simulink model "bluetooth_voice"  (Simulink 4.1.1)
settings: Solver=VariableStepDiscrete  StartTime=0.0  StopTime=2.7  RelTol=1e-3
PreLoadFcn:
  | bluetooth_init;
values from neighbouring files (symbols this model uses):
  Access_Code = zeros(72,1); Access_Code(1:2:72)=1    [bluetooth_init.m]
  ARQ = [1]    [bluetooth_init.m]
  awgn_channel_seed = randseed(2)    [bluetooth_init.m]
  data_seed = randseed(5)    [bluetooth_init.m]
  Flow_Control = [1]    [bluetooth_init.m]
  Input_Fs = 8000    [bluetooth_init.m]
  Num_Slots_Rate = 6    [device_init.m]
  One_Zero_Payload = zeros(240,1)    [bluetooth_init.m]
  Packet_Type = [1 0 1 0]'    [bluetooth_init.m]
  Sequence = [1]    [bluetooth_init.m]
  Slave_Address = [1 0 1]'    [bluetooth_init.m]
  Slot_Enable_Phase = Slot_Pair*2-2    [device_init.m]
  Slot_Ts = (1/1600)    (= 0.000625)    [device_init.m]
  Tx_Ts = Slot_Ts*6    (= 0.00375)    [device_init.m]
undefined symbols (not defined in the file or in its folder): Fs, g, jet
libraries: commblkcod2 x48, dspsrcs3 x25, dspsigops x18, simulink3 x16, dspsigattribs x9, dspbuff3 x7, dspindex x7, bluetooth_lib x5, dspmathops x4, dspsnks3 x4, dspmtrx3 x3, commdigbbndfm2 x3
(part 1 of 2)
settings Model: Creator=Stuart McGarrity  LastModifiedBy=stuartm  SaveTime=off  SaveOutput=off  OptimizeBlockIOStorage=off  BlockReductionOpt=off
settings Model: ModifiedComment=|
  | stuartm -- Fri Jul 20 12:58:27 2001 -- Version 1.201
  | Fix for R12.1. Changed CPM modulator. Replaced enable subsystems in channel with "switch case".
settings Model: ModifiedHistory=|
  | stuartm -- Fri Jul 20 12:58:27 2001 -- Version 1.201
  | Fix for R12.1. Changed CPM modulator. Replaced enable subsystems in channel with "switch case".
  | 
  | 
  | stuartm -- Sun Jul 08 13:59:13 2001 -- Version 1.172
  | Added gain mask at output of transmitter to run it off after 374 bits.
  | 
  | stuartm -- Sun Jul 08 13:53:19 2001 -- Version 1.171
  | Changed hop generator to randint block. Put zero padiing back to before transmitter.
  | 
  | 
  | Started with bluetooth_voice2. Move zero pad from input to output of transmitter. Now only transmits 374 bits
  | 
  | Added channel option

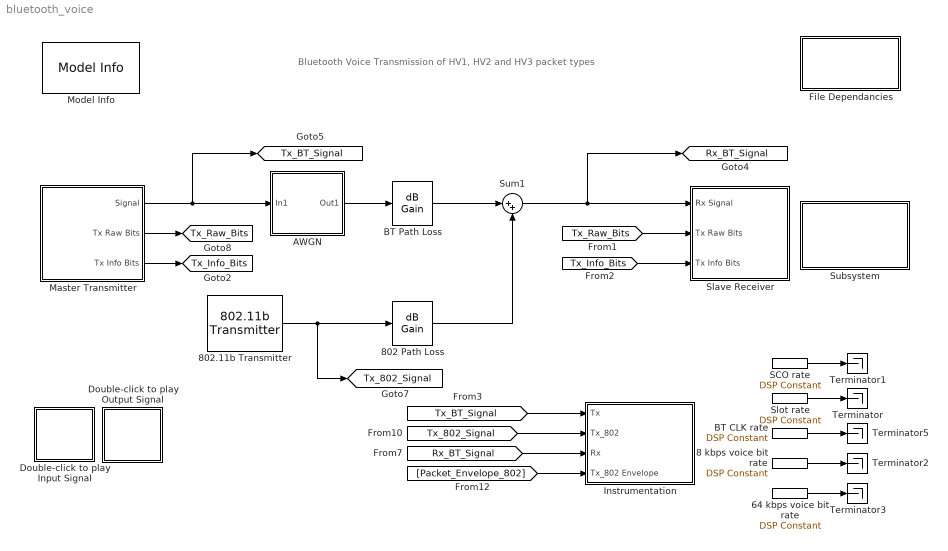
== system bluetooth_voice ==
  note: Bluetooth Voice Transmission
      | of HV1, HV2 and HV3 packet types
  64 kbps voice bit rate : dspsrcs3/DSP Constant  Value=1  InterpretAs1D=off  SampleMode=Discrete  Ts=1/64000  FramebasedOutput=off
  8 kbps voice bit rate : dspsrcs3/DSP Constant  Value=1  InterpretAs1D=off  SampleMode=Discrete  Ts=1/8000  FramebasedOutput=off
  802 Path Loss : dspmathops/dB Gain  Gain=g  dB=-40  intype=Amplitude
  802.11b Transmitter : bluetooth_lib/802.11b Transmitter  On=on  rate=200  m=1e-3  v=0  power=1  Freq_Number=39  rate_seed=rate_802_seed  awgn_seed=awgn_802_seed
  AWGN : Subsystem  TreatAsAtomicUnit=on  mask(Optional channel){AWGN_On=on, EsNo=14, Power=.001, Symbol_Period=1e-6, seed=awgn_channel_seed}
      mask prompts: AWGN_On "Turn on AWGN"; EsNo "Es/No"; Power "Input Power"; Symbol_Period "Symbol Period"
      mask init:
      | if AWGN_On==1
      |    Name='On';
      | else
      |   Name='Off';
      | end;
      settings: RTWFcnNameOpts=Auto  RTWFileNameOpts=Auto
      mask Display: disp(['AWGN is ' Name])
  BT CLK rate : dspsrcs3/DSP Constant  Value=1  InterpretAs1D=off  SampleMode=Discrete  Ts=.5/1600  FramebasedOutput=off
  BT Path Loss : dspmathops/dB Gain  Gain=g  dB=-40  intype=Amplitude
  Double-click to play Input Signal : Subsystem  mask(Plot histogram){}
      mask init:
      | [x,y,x1,y1,x2,y2] = dspblkwao2('icon');
      settings: OpenFcn=[Input_Wave,Input_Fs]=wavread('Input.wav');sound(Input_Wave,Input_Fs);  RTWFcnNameOpts=Auto  RTWFileNameOpts=Auto
      mask Display:
      | patch(x1,y1,[1 1 1]*.5);
      | patch(x2,y2);
      | plot(x,y); plot(x1,y1)
  Double-click to play Output Signal : Subsystem  mask(Plot histogram){}
      mask init:
      | [x,y,x1,y1,x2,y2] = dspblkwao2('icon');
      settings: OpenFcn=[Output_Wave,Output_Fs]=wavread('Output.wav');sound(Output_Wave,Output_Fs);  RTWFcnNameOpts=Auto  RTWFileNameOpts=Auto
      mask Display:
      | patch(x1,y1,[1 1 1]*.5);
      | patch(x2,y2);
      | plot(x,y); plot(x1,y1)
  File Dependancies : Subsystem
      settings: RTWFcnNameOpts=Auto  RTWFileNameOpts=Auto
      mask Display: disp('File\nDependancies')
  Instrumentation : Subsystem  TreatAsAtomicUnit=on  mask(Instrumentation){On=on, Off=off}
      mask init:
      | if strcmp(On,'on')
      |   string='Instrumentation\nis On\n(Double-Click\n to Toggle)\n ';
      |   set_param([gcb,'/State'],'Value','1');
      | else
      |   string='Instrumentation\nis Off\n(Double-Click\n to Toggle)\n ';
      |   set_param([gcb,'/State'],'Value','0');
      | end
      settings: OpenFcn=temp=get_param(gcb,'On');set_param(gcb,'On', get_param(gcb,'Off'));set_param(gcb,'Off', temp);  RTWFcnNameOpts=Auto  RTWFileNameOpts=Auto
      mask Display: disp(string);
  Master Transmitter : Subsystem  mask(Master Transmitter){HV_Type=HV3, Slot_Pair=1&2}
      mask prompts: HV_Type "HV Packet Type"; Slot_Pair "Initial Slot Pair for HV2 or HV3"
      mask init:
      | device_init
      settings: RTWFcnNameOpts=Auto  RTWFileNameOpts=Auto
      mask StyleString: popup(HV1|HV2|HV3),popup(1&2|3&4|5&6)
      mask Display: plot(0,0,100,100,[30,60,60,55,55,30,30],[10,10,90,90,70,70,10],[35,35,55,55,35],[64,45,45,64,64])
  Model Info : simulink3/Signals & Systems/Model Info  InitialBlockCM=none  BlockCM=none  Frame=on  DisplayStringWithTags=|  HorizontalTextAlignment=Center  LeftAlignmentValue=0.5  SourceBlockDiagram=bluetooth_voice  TagMaxNumber=20
      | Bluetooth Voice
      | %<ModelVersion>
  SCO rate : dspsrcs3/DSP Constant  Value=1  InterpretAs1D=off  SampleMode=Discrete  Ts=6/1600  FramebasedOutput=off
  Slave Receiver : Subsystem  mask(Slave Receiver){HV_Type=HV3, Slot_Pair=1&2}
      mask prompts: HV_Type "HV Packet Type"; Slot_Pair "Initial Slot Pair for HV2 or HV3"
      mask init:
      | device_init
      settings: RTWFcnNameOpts=Auto  RTWFileNameOpts=Auto
      mask StyleString: popup(HV1|HV2|HV3),popup(1&2|3&4|5&6)
      mask Display: plot(15,5,95,80,[26, 28,35,44,58,85,87,92,86,59,46,46,38, 31, 27,26],[55,49,45,45,34,15,10,16,17,37,50,58,66,67,62,55],[32,34,37,42,46,46],[67,69,71,70,66,58],[27,25,24,21,23,26],[52,49,45,47,52,58],[35,38,40,42,44],[66,67,66,64,61],[34,32,38,40,34],[60,56,51,55,60])
  Slot rate : dspsrcs3/DSP Constant  Value=1  InterpretAs1D=off  SampleMode=Discrete  Ts=1/1600  FramebasedOutput=off
  Subsystem : Subsystem
      settings: OpenFcn=open_system([bdroot '/Slave Receiver/Demodulate and decode'])  RTWFcnNameOpts=Auto  RTWFileNameOpts=Auto
      mask Display: disp('Double-click to open\n subsystem with\nBER meters\ninside receiver')
  Sum1 : Sum  Inputs=|++  SaturateOnIntegerOverflow=on
  Terminator{,1..3,5} (5 alike) : Terminator
  tag scope: Rx_BT_Signal=global, Tx_802_Signal=global, Tx_BT_Signal=global, Tx_Info_Bits=global, Tx_Raw_Bits=global
  wires:
  Master Transmitter/1(Signal) -> [Tx_BT_Signal], AWGN/1(In1)
  Sum1/1 -> [Rx_BT_Signal], Slave Receiver/1(Rx Signal)
  Master Transmitter/2(Tx Raw Bits) -> [Tx_Raw_Bits]
  Slot rate/1 -> Terminator/1
  SCO rate/1 -> Terminator1/1
  [Tx_Raw_Bits] -> Slave Receiver/2(Tx Raw Bits)
  64 kbps voice bit rate/1 -> Terminator3/1
  BT CLK rate/1 -> Terminator5/1
  Master Transmitter/3(Tx Info Bits) -> [Tx_Info_Bits]
  [Tx_Info_Bits] -> Slave Receiver/3(Tx Info Bits)
  8 kbps voice bit rate/1 -> Terminator2/1
  802.11b Transmitter/1 -> [Tx_802_Signal], 802 Path Loss/1
  802 Path Loss/1 -> Sum1/2
  AWGN/1(Out1) -> BT Path Loss/1
  BT Path Loss/1 -> Sum1/1
  [Tx_BT_Signal] -> Instrumentation/1(Tx)
  [Rx_BT_Signal] -> Instrumentation/3(Rx)
  [Tx_802_Signal] -> Instrumentation/2(Tx_802)
  [Packet_Envelope_802] -> Instrumentation/4(Tx_802 Envelope)

== system bluetooth_voice/AWGN ==
  In1 : Inport  Port=1  LatchInput=off
  Generate noise only for slot 1 : simulink3/Nonlinear/Manual Switch  sw=0  action=0
  Mode : Constant  Value=AWGN_On
  Slot 1 enable2 : dspsrcs3/Signal From Workspace  X=[1 0 0 0 0 0]  Ts=625e-6  nsamps=1  OutputAfterFinalValue=Cyclic Repetition
  Slot 1 enable3 : dspsrcs3/Signal From Workspace  X=[1 1 1 1 1 1 ]  Ts=625e-6  nsamps=1  OutputAfterFinalValue=Cyclic Repetition
  Subsystem : Subsystem  TreatAsAtomicUnit=on
      settings: RTWFcnNameOpts=Auto  RTWFileNameOpts=Auto
  Out1 : Outport  Port=1  InitialOutput=0
  wires:
  Mode/1 -> Subsystem/1(In1)
  Subsystem/1(Out1) -> Out1/1
  Slot 1 enable3/1 -> Generate noise only for slot 1/2
  Generate noise only for slot 1/1 -> Subsystem/Enable
  Slot 1 enable2/1 -> Generate noise only for slot 1/1
  In1/1 -> Subsystem/2(In2)

== system bluetooth_voice/Double-click to play Input Signal ==

== system bluetooth_voice/Double-click to play Output Signal ==

== system bluetooth_voice/File Dependancies ==
  note: * bluetooth_init.m: Workspace initialization routine called by PreLoadFcn
      | * device_init.m: Transmitter and receiver mask initialization function
      | * bluetooth_lib.mld: Simuink library containing 802.11b transmitter, BT hop generator and BT clock
      | * poiss_gaus_pr3.m: Variable time-step M Code S-function to generate 802.11b possion packets
      | * scondemohecgen.c: S-Function builder source for HEC
      | * scondemohecgen.dll: S-Function builder DLL
      | * scondemohecgen_wrapper.c: S-Function support file
      | * Input.wav: Input wave file
      | * Output.wav: Output wave file
  note: File dependancies: These files need to on MATLAB path

== system bluetooth_voice/Instrumentation ==
  Tx : Inport  Port=1  LatchInput=off
  Tx_802 : Inport  Port=2  LatchInput=off
  Rx : Inport  Port=3  LatchInput=off
  Tx_802 Envelope : Inport  Port=4  LatchInput=off
  802.11 Packets  Transmitted : Display
      settings: Format=short
  Counter : dspswit3/Counter  Direction=Up  CountEvent=Rising edge  CounterSize=User defined  MaxCount=1000  InitialCount=0  Output=Count  HitValue=32  ResetInput=off  SamplesPerFrame=1  Ts=1
  State : Constant  Value=1
  Subsystem : Subsystem  TreatAsAtomicUnit=on
      settings: RTWFcnNameOpts=Auto  RTWFileNameOpts=Auto
  To Workspace : ToWorkspace  VariableName=Num_802_packets  SampleTime=-1  SaveFormat=Array
      settings: MaxDataPoints=1
  wires:
  Counter/1 -> To Workspace/1, 802.11 Packets  Transmitted/1
  State/1 -> Subsystem/Enable
  Tx_802 Envelope/1 -> Counter/1
  Tx_802/1 -> Subsystem/2(In2)
  Tx/1 -> Subsystem/1(In1)
  Rx/1 -> Subsystem/3(In3)

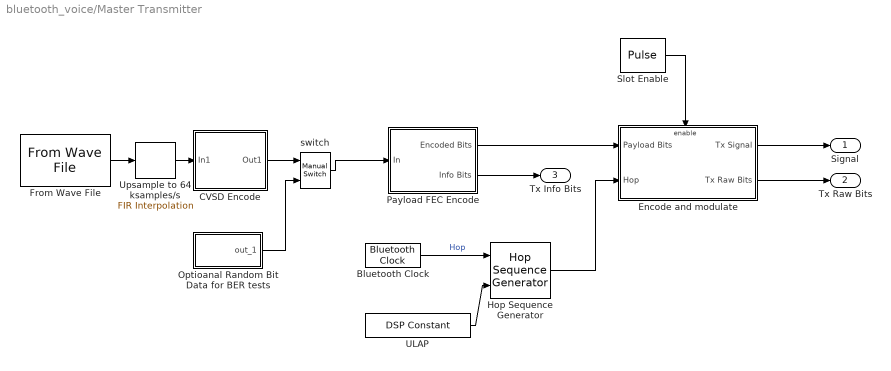
== system bluetooth_voice/Master Transmitter ==
  Bluetooth Clock : bluetooth_lib/Bluetooth Clock  Ts=(1/1600)/2
  CVSD Encode : Subsystem  mask(CVSD Encoder){min_step=10, max_step=1280, accum_decay=1-1/32, step_decay=1-1/1024}
      mask prompts: min_step "Minimum Step Size"; max_step "Maximum Step Size"; accum_decay "Accumulator Decay"; step_decay "Step Decay"
      mask help: Encode a 64 K samples per sec speech signal into a 64Kbps bit stream.
      mask init:
      | pos_accum_max = 2^15 - 1;
      | neg_accum_max = -2^15 + 1;
      settings: RTWFcnNameOpts=Auto  RTWFileNameOpts=Auto
      mask Display: disp('CVSD\nEncode')
  Encode and modulate : Subsystem  TreatAsAtomicUnit=on
      settings: RTWFcnNameOpts=Auto  RTWFileNameOpts=Auto
  From Wave File : dspsrcs3/From Wave File  FileName=Input.wav  SamplesPerFrame=1  MinBufSize=256
  Hop Sequence Generator : bluetooth_lib/Hop Sequence Generator  Hop_Mode=Connection State Hop Sequence  hop_seed=hop_seed  fixed_hop_freq=fixed_hop_freq
  Optioanal Random Bit Data for BER tests : Subsystem  mask(Random-Integer Generator){mul=2, seed=data_seed, Ts=1/64000, frameBased=off, sampPerFrame=1, orient=off}
      mask prompts: mul "M-ary number:"; seed "Initial seed:"; Ts "Sample time:"; frameBased "Frame-based outputs"; sampPerFrame "Samples per frame:"; orient "Interpret vector parameters as 1-D"
      mask help: Generate integers randomly distributed in range [0, M-1], where M is the M-ary number.
      mask init:
      | if (frameBased & sampPerFrame > 1), dsp_sampFrame = sampPerFrame;
      | else dsp_sampFrame = 1; end
      | eStr=commblkrandintsrc2(gcb,'init');
      | if(eStr.ecode==1)
      |     error(eStr.emsg);
      | end
      settings: RTWFcnNameOpts=Auto  RTWFileNameOpts=Auto
      mask Help: helpview(commbhelp)
      mask CallbackString: |||commblkrandintsrc2(gcb,'cbFrameBased');||commblkrandintsrc2(gcb,'cbOrient');
      mask Display: disp('Random bits')
  Payload FEC Encode : Subsystem
      settings: RTWFcnNameOpts=Auto  RTWFileNameOpts=Auto
  Slot Enable : DiscretePulseGenerator  PulseType=Sample-based  Amplitude=1  Period=Num_Slots_Rate  PulseWidth=1  PhaseDelay=Slot_Enable_Phase  SampleTime=Slot_Ts
  ULAP : dspsrcs3/DSP Constant  Value=hex2dec('2a96ef25')  InterpretAs1D=off  SampleMode=Discrete  Ts=(1/1600)/2  FramebasedOutput=off
  Upsample to 64 ksamples/s : dspmlti3/FIR Interpolation  h=interp_coeffs  L=8  framing=Maintain input frame size  outputBufInitCond=0
  switch : simulink3/Nonlinear/Manual Switch  sw=1  action=0
  Signal : Outport  Port=1
  Tx Raw Bits : Outport  Port=2
  Tx Info Bits : Outport  Port=3
  wires:
  Slot Enable/1 -> Encode and modulate/Enable
  Encode and modulate/1(Tx Signal) -> Signal/1
  Payload FEC Encode/1(Encoded Bits) -> Encode and modulate/1(Payload Bits)
  From Wave File/1 -> Upsample to 64 ksamples/s/1
  Upsample to 64 ksamples/s/1 -> CVSD Encode/1(In1)
  Payload FEC Encode/2(Info Bits) -> Tx Info Bits/1
  Encode and modulate/2(Tx Raw Bits) -> Tx Raw Bits/1
  Hop Sequence Generator/1 -> Encode and modulate/2(Hop)
  ULAP/1 -> Hop Sequence Generator/2
  Bluetooth Clock/1 -> Hop Sequence Generator/1  "Hop"
  Optioanal Random Bit Data for BER tests/1(out_1) -> switch/2
  CVSD Encode/1(Out1) -> switch/1
  switch/1 -> Payload FEC Encode/1(In)

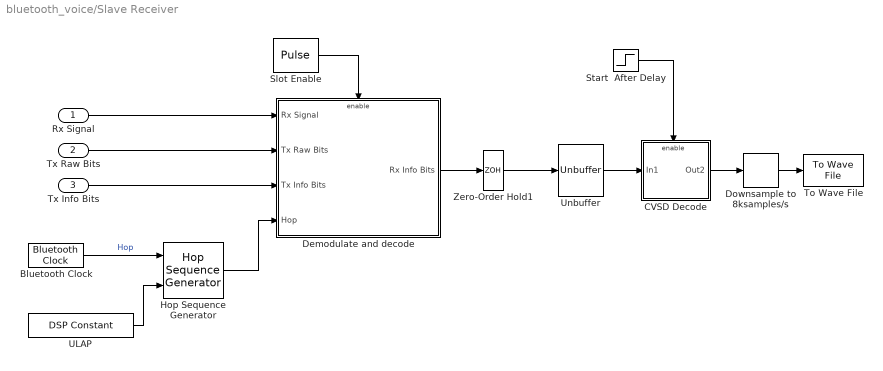
== system bluetooth_voice/Slave Receiver ==
  Rx Signal : Inport  Port=1  LatchInput=off
  Tx Raw Bits : Inport  Port=2  LatchInput=off
  Tx Info Bits : Inport  Port=3  LatchInput=off
  Bluetooth Clock : bluetooth_lib/Bluetooth Clock  Ts=(1/1600)/2
  CVSD Decode : Subsystem  TreatAsAtomicUnit=on  mask(CVSD Decoder){min_step=10, max_step=1280, accum_decay=1-1/32, step_decay=1-1/1024}
      mask prompts: min_step "Minimum Step Size"; max_step "Maximum Step Size"; accum_decay "Accumulator Decay"; step_decay "Step Decay"
      mask init:
      | pos_accum_max = 2^15 - 1;
      | neg_accum_max = -2^15 + 1;
      settings: RTWFcnNameOpts=Auto  RTWFileNameOpts=Auto
      mask Display: disp('CVSD\nDecoder')
  Demodulate and decode : Subsystem  TreatAsAtomicUnit=on
      settings: RTWFcnNameOpts=Auto  RTWFileNameOpts=Auto
  Downsample to 8ksamples/s : dspsigops/Downsample  N=8  phase=0  ic=0  smode=Allow multirate  fmode=Maintain input frame size
  Hop Sequence Generator : bluetooth_lib/Hop Sequence Generator  Hop_Mode=Connection State Hop Sequence  hop_seed=hop_seed  fixed_hop_freq=fixed_hop_freq
  Slot Enable : DiscretePulseGenerator  PulseType=Sample-based  Amplitude=1  Period=Num_Slots_Rate  PulseWidth=1  PhaseDelay=Slot_Enable_Phase  SampleTime=Slot_Ts
  Start  After Delay : Step  Time=0.01  Before=0  After=1  SampleTime=1/64000
  To Wave File : dspsnks3/To Wave File  filename=Output  sampleWidth=8  MinNumSamples=256
  ULAP : dspsrcs3/DSP Constant  Value=hex2dec('2a96ef25')  InterpretAs1D=off  SampleMode=Discrete  Ts=(1/1600)/2  FramebasedOutput=off
  Unbuffer : dspbuff3/Unbuffer  ic=0
  Zero-Order Hold1 : ZeroOrderHold  SampleTime=Tx_Ts
  wires:
  Slot Enable/1 -> Demodulate and decode/Enable
  Rx Signal/1 -> Demodulate and decode/1(Rx Signal)
  Tx Raw Bits/1 -> Demodulate and decode/2(Tx Raw Bits)
  CVSD Decode/1(Out2) -> Downsample to 8ksamples/s/1
  Demodulate and decode/1(Rx Info Bits) -> Zero-Order Hold1/1
  ULAP/1 -> Hop Sequence Generator/2
  Bluetooth Clock/1 -> Hop Sequence Generator/1  "Hop"
  Hop Sequence Generator/1 -> Demodulate and decode/4(Hop)
  Zero-Order Hold1/1 -> Unbuffer/1
  Downsample to 8ksamples/s/1 -> To Wave File/1
  Start  After Delay/1 -> CVSD Decode/Enable
  Unbuffer/1 -> CVSD Decode/1(In1)
  Tx Info Bits/1 -> Demodulate and decode/3(Tx Info Bits)

== system bluetooth_voice/Subsystem ==

== system bluetooth_voice/AWGN/Subsystem ==
  In1 : Inport  Port=1  LatchInput=off
  In2 : Inport  Port=2  LatchInput=off
  Enable : EnablePort
  Add noise : Subsystem  TreatAsAtomicUnit=on
      settings: RTWFcnNameOpts=Auto  RTWFileNameOpts=Auto
  If : If  NumInputs=1  IfExpression=u1 == 0  ShowElse=on
  Merge : Merge  Inputs=2  AllowUnequalInputPortWidths=off  InputPortOffsets=[]
  Pass Through : Subsystem  TreatAsAtomicUnit=on
      settings: RTWFcnNameOpts=Auto  RTWFileNameOpts=Auto
  Out1 : Outport  Port=1
  wires:
  Add noise/1(Out1) -> Merge/2
  Pass Through/1(Out1) -> Merge/1
  If/1 -> Pass Through/Action
  In2/1 -> Pass Through/1(In1), Add noise/1(In1)
  If/2 -> Add noise/Action
  In1/1 -> If/1
  Merge/1 -> Out1/1

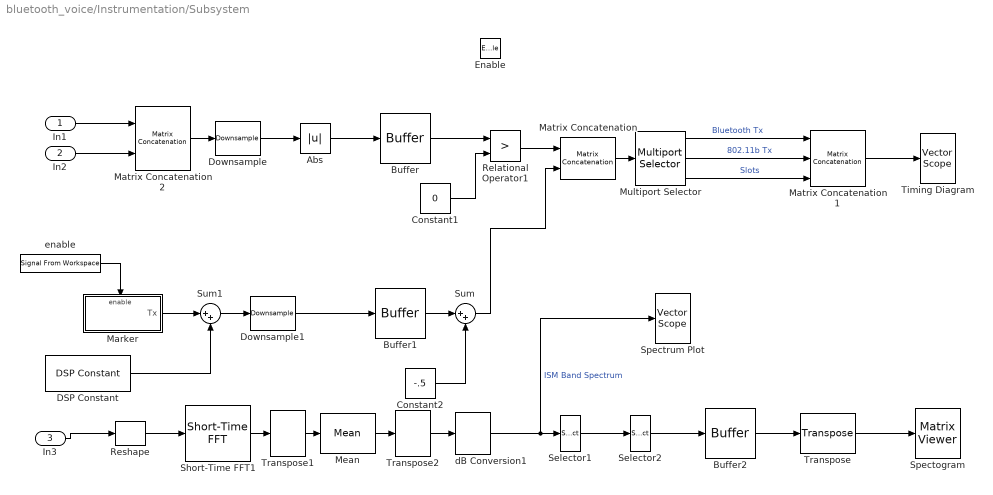
== system bluetooth_voice/Instrumentation/Subsystem ==
  In1 : Inport  Port=1  LatchInput=off
  In2 : Inport  Port=2  LatchInput=off
  In3 : Inport  Port=3  LatchInput=off
  Enable : EnablePort
  Abs : Abs  SaturateOnIntegerOverflow=on
  Buffer : dspbuff3/Buffer  N=60*500  V=59*500  ic=0
  Buffer1 : dspbuff3/Buffer  N=60*500  V=59*500  ic=0
  Buffer2 : dspbuff3/Buffer  N=60  V=59  ic=-70
  Constant1 : Constant  Value=0
  Constant2 : Constant  Value=-.5
  DSP Constant : dspsrcs3/DSP Constant  Value=.2*[ones(1,36600) zeros(1,62500-36600)]'  InterpretAs1D=off  SampleMode=Discrete  Ts=625e-6  FramebasedOutput=on
  Downsample : dspsigops/Downsample  N=125  phase=0  ic=0  smode=Allow multirate  fmode=Maintain input frame rate
  Downsample1 : dspsigops/Downsample  N=125  phase=0  ic=0  smode=Allow multirate  fmode=Maintain input frame rate
  Marker : Subsystem  TreatAsAtomicUnit=on
      settings: RTWFcnNameOpts=Auto  RTWFileNameOpts=Auto
  Matrix Concatenation : simulink3/Signals & Systems/Matrix Concatenation  numInports=2  catMethod=Horizontal
  Matrix Concatenation1 : simulink3/Signals & Systems/Matrix Concatenation  numInports=3  catMethod=Horizontal
  Matrix Concatenation2 : simulink3/Signals & Systems/Matrix Concatenation  numInports=2  catMethod=Horizontal
  Mean : dspstat3/Mean  run=off  reset_popup=None
  Multiport Selector : dspindex/Multiport Selector  rowsOrCols=Columns  idxCellArray={ 1,2,3}  idxErrMode=Clip Index
  Relational Operator1 : RelationalOperator  Operator=>
  Reshape : simulink3/Signals & Systems/Reshape  OutputDimensionality=Customize  OutputDimensions=[500,125]
  Selector1 : Selector  InputType=Vector  ElementSrc=Internal  Elements=[257:512 1:256]  RowSrc=Internal  Rows=1  ColumnSrc=Internal  Columns=1  InputPortWidth=512
  Selector2 : Selector  InputType=Vector  ElementSrc=Internal  Elements=7:506  RowSrc=Internal  Rows=1  ColumnSrc=Internal  Columns=1  InputPortWidth=512
  Short-Time FFT1 : dspspect3/Short-Time FFT  wintype=Hanning  Rs=50  beta=5  winsamp=Periodic  inheritFFT=off  fftsize=512  navg=1
  Spectogram : dspsnks3/Matrix Viewer  ImageParams=on  CMapStr=jet(256)  AxisColorbar=on  AxisParams=on  AxisOrigin=Lower left corner  XLabel=Time Index  YLabel=Frequency Index  ZLabel=dB Magnitude  FigPos=[65 269 688 127]  AxisZoom=on
      settings: YMin=-60  YMax=-30
  Spectrum Plot : dspsnks3/Vector Scope  ScopeProperties=on  Domain=Frequency  HorizSpan=1  DisplayProperties=off  AxisGrid=on  Memory=off  FrameNumber=on  AxisLegend=on  AxisZoom=off  OpenScopeAtSimStart=on  OpenScopeImmediately=off  FigPos=[2 605 774 120]  AxisProperties=off  XUnits=Hertz  XRange=[-Fs/2...Fs/2]  InheritXIncr=off  XIncr=1e-8  XLabel=Time  YUnits=Magnitude  YLabel=Magnitude, dB  LineProperties=off  LineStyles=--
      settings: YMin=-80.906815143504  YMax=-25.7732682054945
  Sum : Sum  Inputs=|++  SaturateOnIntegerOverflow=on
  Sum1 : Sum  Inputs=|++  SaturateOnIntegerOverflow=on
  Timing Diagram : dspsnks3/Vector Scope  ScopeProperties=on  Domain=User-defined  HorizSpan=1  DisplayProperties=off  AxisGrid=on  Memory=off  FrameNumber=on  AxisLegend=on  AxisZoom=off  OpenScopeAtSimStart=on  OpenScopeImmediately=off  FigPos=[8 427 776 129]  AxisProperties=off  XUnits=Hertz  XRange=[0...Fs/2]  InheritXIncr=off  XIncr=125*1e-8  XLabel=Time (s)  YUnits=dB  YLabel=Amplitude  LineProperties=off  LineStyles=-|-  LineColors=[0 1 0]|[1 0 0]
      settings: YMin=-0.525  YMax=1.05
  Transpose : dspmtrx3/Transpose  Hermitian=off
  Transpose1 : dspmtrx3/Transpose  Hermitian=off
  Transpose2 : dspmtrx3/Transpose  Hermitian=off
  dB Conversion1 : dspmathops/dB Conversion  dBtype=dB  intype=Power  R=1  fuzz=on
  enable : dspsrcs3/Signal From Workspace  X=[1 0 0 0 0 0]  Ts=625e-6  nsamps=1  OutputAfterFinalValue=Cyclic Repetition
  wires:
  DSP Constant/1 -> Sum1/2
  Sum1/1 -> Downsample1/1
  Marker/1(Tx) -> Sum1/1
  Buffer1/1 -> Sum/1
  Constant2/1 -> Sum/2
  Matrix Concatenation/1 -> Multiport Selector/1
  Relational Operator1/1 -> Matrix Concatenation/1
  Sum/1 -> Matrix Concatenation/2
  Downsample1/1 -> Buffer1/1
  Multiport Selector/3 -> Matrix Concatenation1/3  "Slots"
  enable/1 -> Marker/Enable
  Multiport Selector/2 -> Matrix Concatenation1/2  "802.11b Tx"
  Multiport Selector/1 -> Matrix Concatenation1/1  "Bluetooth Tx"
  Matrix Concatenation2/1 -> Downsample/1
  In1/1 -> Matrix Concatenation2/1
  In2/1 -> Matrix Concatenation2/2
  Buffer/1 -> Relational Operator1/1
  Constant1/1 -> Relational Operator1/2
  Transpose2/1 -> dB Conversion1/1
  Transpose1/1 -> Mean/1
  Mean/1 -> Transpose2/1
  Reshape/1 -> Short-Time FFT1/1
  In3/1 -> Reshape/1
  Matrix Concatenation1/1 -> Timing Diagram/1
  Selector2/1 -> Buffer2/1
  Selector1/1 -> Selector2/1
  Short-Time FFT1/1 -> Transpose1/1
  dB Conversion1/1 -> Spectrum Plot/1, Selector1/1  "ISM Band Spectrum"
  Downsample/1 -> Abs/1
  Abs/1 -> Buffer/1
  Buffer2/1 -> Transpose/1
  Transpose/1 -> Spectogram/1

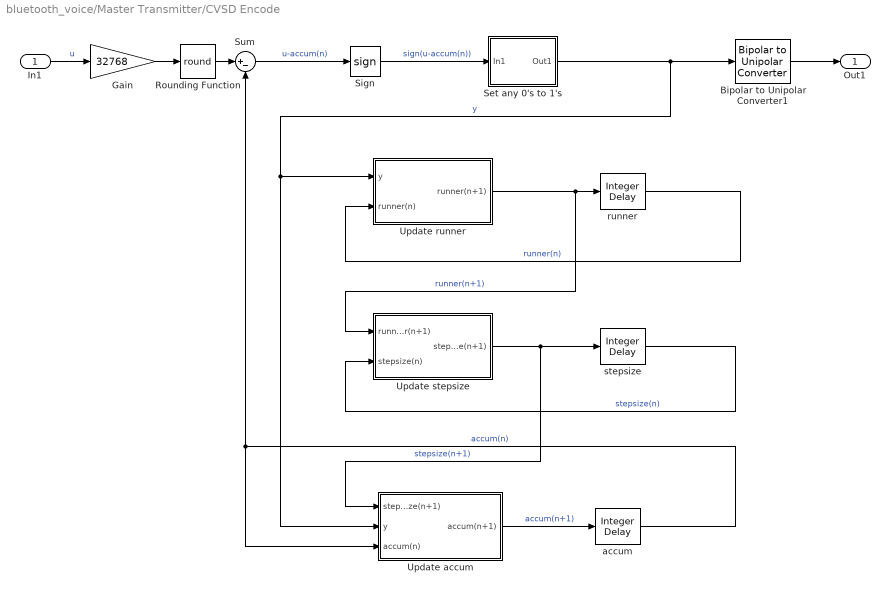
== system bluetooth_voice/Master Transmitter/CVSD Encode ==
  In1 : Inport  Port=1  LatchInput=off
  Bipolar to Unipolar Converter1 : commutil2/Bipolar to Unipolar Converter  M=2  polarity=Negative
  Gain : Gain  Gain=32768  Multiplication=Element-wise(K.*u)  SaturateOnIntegerOverflow=on
  Rounding Function : Rounding  Operator=round
  Set any 0's to 1's : Subsystem
      settings: RTWFcnNameOpts=Auto  RTWFileNameOpts=Auto
  Sign : Signum
  Sum : Sum  Inputs=|+-  SaturateOnIntegerOverflow=on
  Update accum : Subsystem
      settings: RTWFcnNameOpts=Auto  RTWFileNameOpts=Auto
  Update runner : Subsystem
      settings: RTWFcnNameOpts=Auto  RTWFileNameOpts=Auto
  Update stepsize : Subsystem
      settings: RTWFcnNameOpts=Auto  RTWFileNameOpts=Auto
  accum : dspsigops/Integer Delay  delay=1  ic=0
  runner : dspsigops/Integer Delay  delay=1  ic=10
  stepsize : dspsigops/Integer Delay  delay=1  ic=min_step
  Out1 : Outport  Port=1
  wires:
  Gain/1 -> Rounding Function/1
  Rounding Function/1 -> Sum/1
  Bipolar to Unipolar Converter1/1 -> Out1/1
  In1/1 -> Gain/1  "u"
  Sum/1 -> Sign/1  "u-accum(n)"
  accum/1 -> Sum/2, Update accum/3(accum(n))  "accum(n)"
  Set any 0's to 1's/1(Out1) -> Bipolar to Unipolar Converter1/1, Update runner/1(y), Update accum/2(y)  "y"
  runner/1 -> Update runner/2(runner(n))  "runner(n)"
  Update runner/1(runner(n+1)) -> runner/1, Update stepsize/1(runner(n+1))  "runner(n+1)"
  Sign/1 -> Set any 0's to 1's/1(In1)  "sign(u-accum(n))"
  stepsize/1 -> Update stepsize/2(stepsize(n))  "stepsize(n)"
  Update stepsize/1(stepsize(n+1)) -> stepsize/1, Update accum/1(stepsize(n+1))  "stepsize(n+1)"
  Update accum/1(accum(n+1)) -> accum/1  "accum(n+1)"

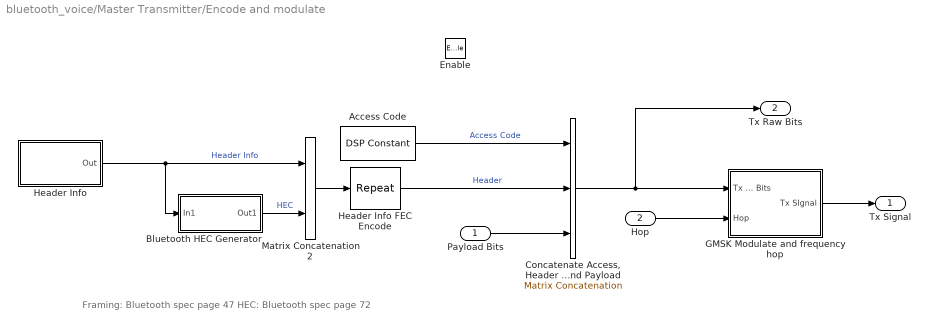
== system bluetooth_voice/Master Transmitter/Encode and modulate ==
  note: Framing: Bluetooth spec page 47
      | HEC: Bluetooth spec page 72
  Payload Bits : Inport  Port=1  LatchInput=off  SampleTime=625e-6
  Hop : Inport  Port=2  LatchInput=off  SampleTime=625e-6
  Enable : EnablePort
  Access Code : dspsrcs3/DSP Constant  Value=Access_Code  InterpretAs1D=off  SampleMode=Discrete  Ts=Slot_Ts  FramebasedOutput=on
  Bluetooth HEC Generator : Subsystem  mask(Bluetooth HEC Generator){uap=[1 0 0 1 0 1 1 0]}
      mask help: Compute the Bluetooth Header Error Check (HEC) as specified in section 5.4 of the Bluetooth specification. The Upper Address Part (UAP) is used to initialize the state of the encoder. The UAP is an 8-bit vector, LSB first.
      settings: RTWFcnNameOpts=Auto  RTWFileNameOpts=Auto
      mask Display: disp('Bluetooth\nHEC Generator')
  "Concatenate Access, Header and Payload" : simulink3/Signals & Systems/Matrix Concatenation  numInports=3  catMethod=Vertical
  GMSK Modulate and frequency hop : Subsystem
      settings: RTWFcnNameOpts=Auto  RTWFileNameOpts=Auto
  Header Info : Subsystem
      settings: RTWFcnNameOpts=Auto  RTWFileNameOpts=Auto
      mask Display: disp('Header Info')
  Header Info FEC Encode : dspsigops/Repeat  N=3  ic=0  mode=Maintain input frame rate
  Matrix Concatenation2 : simulink3/Signals & Systems/Matrix Concatenation  numInports=2  catMethod=Vertical
  Tx Signal : Outport  Port=1  OutputWhenDisabled=reset  InitialOutput=0
  Tx Raw Bits : Outport  Port=2  OutputWhenDisabled=reset  InitialOutput=0
  wires:
  GMSK Modulate and frequency hop/1(Tx SIgnal) -> Tx Signal/1
  "Concatenate Access, Header and Payload"/1 -> GMSK Modulate and frequency hop/1(Tx Raw Bits), Tx Raw Bits/1
  Matrix Concatenation2/1 -> Header Info FEC Encode/1
  Bluetooth HEC Generator/1(Out1) -> Matrix Concatenation2/2  "HEC"
  Header Info/1(Out) -> Bluetooth HEC Generator/1(In1), Matrix Concatenation2/1  "Header Info"
  Header Info FEC Encode/1 -> "Concatenate Access, Header and Payload"/2  "Header"
  Access Code/1 -> "Concatenate Access, Header and Payload"/1  "Access Code"
  Payload Bits/1 -> "Concatenate Access, Header and Payload"/3
  Hop/1 -> GMSK Modulate and frequency hop/2(Hop)

== system bluetooth_voice/Master Transmitter/Optioanal Random Bit Data for BER tests ==
  Frame Status Conversion : dspsigattribs/Frame Status Conversion  growRefPort=off  outframe=Sample-based
  Random Source : dspsrcs3/Random Source  SrcType=Uniform  Min=-1+eps  Max=mul-1  Mean=0  Var=1  RepMode=Specify seed  Seed=seed  Inherit=off  SampMode=Discrete  SampTime=Ts  SampFrame=dsp_sampFrame  OutComplex=Real
  Reshape : simulink3/Signals & Systems/Reshape  OutputDimensionality=1-D array  OutputDimensions=[sampPerFrame,max([length(mul), length(seed)])]
  Rounding Function : Rounding  Operator=ceil
  out_1 : Outport  Port=1  InitialOutput=0
  wires:
  Frame Status Conversion/1 -> Reshape/1
  Random Source/1 -> Rounding Function/1
  Reshape/1 -> out_1/1
  Rounding Function/1 -> Frame Status Conversion/1

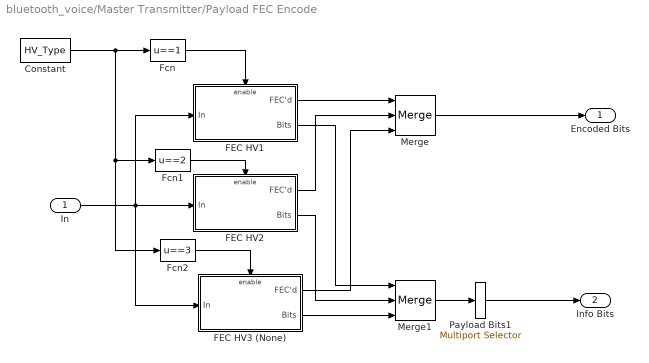
== system bluetooth_voice/Master Transmitter/Payload FEC Encode ==
  In : Inport  Port=1  LatchInput=off
  Constant : Constant  Value=HV_Type
  FEC HV1 : Subsystem  TreatAsAtomicUnit=on
      settings: RTWFcnNameOpts=Auto  RTWFileNameOpts=Auto
  FEC HV2 : Subsystem  TreatAsAtomicUnit=on
      settings: RTWFcnNameOpts=Auto  RTWFileNameOpts=Auto
  FEC HV3 (None) : Subsystem  TreatAsAtomicUnit=on
      settings: RTWFcnNameOpts=Auto  RTWFileNameOpts=Auto
  Fcn : Fcn  Expr=u==1
  Fcn1 : Fcn  Expr=u==2
  Fcn2 : Fcn  Expr=u==3
  Merge : Merge  Inputs=3  AllowUnequalInputPortWidths=off  InputPortOffsets=[]
  Merge1 : Merge  Inputs=3  AllowUnequalInputPortWidths=off  InputPortOffsets=[]
  Payload Bits1 : dspindex/Multiport Selector  rowsOrCols=Rows  idxCellArray={1:Num_Payload_Bits}  idxErrMode=Clip Index
  Encoded Bits : Outport  Port=1
  Info Bits : Outport  Port=2
  wires:
  In/1 -> FEC HV2/1(In), FEC HV1/1(In), FEC HV3 (None)/1(In)
  Constant/1 -> Fcn/1, Fcn1/1, Fcn2/1
  Fcn/1 -> FEC HV1/Enable
  Fcn1/1 -> FEC HV2/Enable
  Fcn2/1 -> FEC HV3 (None)/Enable
  FEC HV2/1(FEC'd) -> Merge/2
  FEC HV1/2(Bits) -> Merge1/1
  FEC HV2/2(Bits) -> Merge1/2
  FEC HV1/1(FEC'd) -> Merge/1
  Merge/1 -> Encoded Bits/1
  Merge1/1 -> Payload Bits1/1
  FEC HV3 (None)/1(FEC'd) -> Merge/3
  FEC HV3 (None)/2(Bits) -> Merge1/3
  Payload Bits1/1 -> Info Bits/1

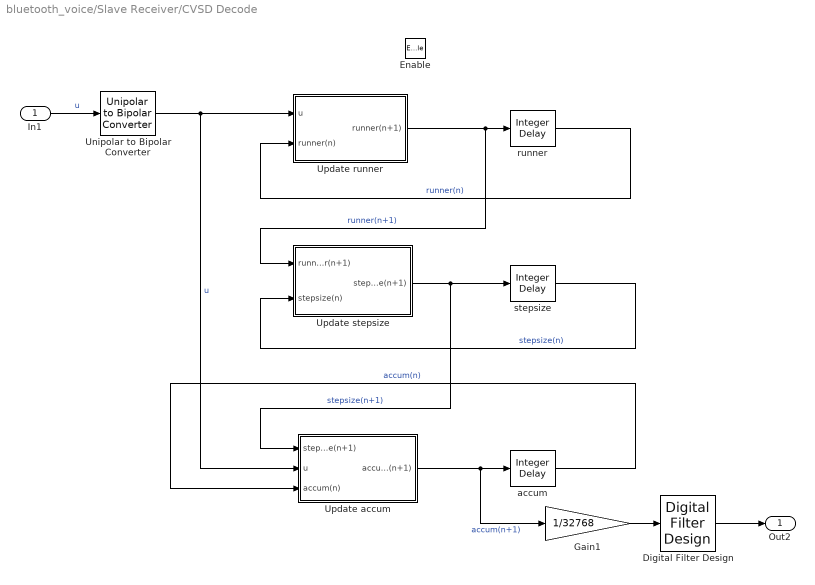
== system bluetooth_voice/Slave Receiver/CVSD Decode ==
  In1 : Inport  Port=1  LatchInput=off
  Enable : EnablePort
  Digital Filter Design : dsparch3/Digital Filter Design
  Gain1 : Gain  Gain=1/32768  Multiplication=Element-wise(K.*u)  SaturateOnIntegerOverflow=on
  Unipolar to Bipolar Converter : commutil2/Unipolar to Bipolar Converter  M=2  polarity=Negative
  Update accum : Subsystem
      settings: RTWFcnNameOpts=Auto  RTWFileNameOpts=Auto
  Update runner : Subsystem
      settings: RTWFcnNameOpts=Auto  RTWFileNameOpts=Auto
  Update stepsize : Subsystem
      settings: RTWFcnNameOpts=Auto  RTWFileNameOpts=Auto
  accum : dspsigops/Integer Delay  delay=1  ic=0
  runner : dspsigops/Integer Delay  delay=1  ic=10
  stepsize : dspsigops/Integer Delay  delay=1  ic=min_step
  Out2 : Outport  Port=1
  wires:
  In1/1 -> Unipolar to Bipolar Converter/1  "u"
  accum/1 -> Update accum/3(accum(n))  "accum(n)"
  runner/1 -> Update runner/2(runner(n))  "runner(n)"
  Update runner/1(runner(n+1)) -> runner/1, Update stepsize/1(runner(n+1))  "runner(n+1)"
  stepsize/1 -> Update stepsize/2(stepsize(n))  "stepsize(n)"
  Update stepsize/1(stepsize(n+1)) -> stepsize/1, Update accum/1(stepsize(n+1))  "stepsize(n+1)"
  Update accum/1(accum(n+1)) -> accum/1, Gain1/1  "accum(n+1)"
  Unipolar to Bipolar Converter/1 -> Update accum/2(u), Update runner/1(u)  "u"
  Digital Filter Design/1 -> Out2/1
  Gain1/1 -> Digital Filter Design/1

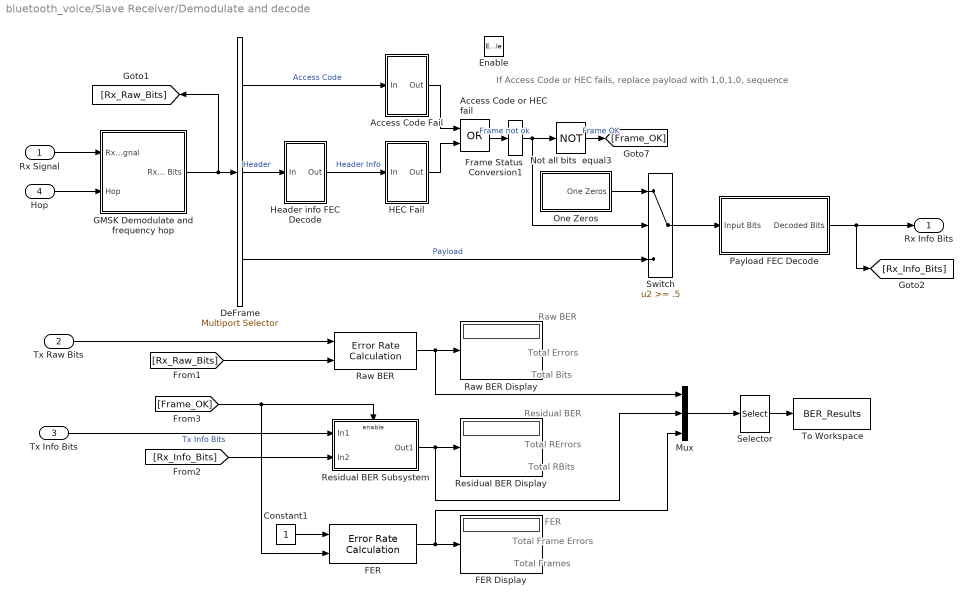
== system bluetooth_voice/Slave Receiver/Demodulate and decode ==
  note: If Access Code or HEC fails,
      | replace payload with 1,0,1,0, sequence
  note: Total Errors
  note: Total Bits
  note: Raw BER
  note: Total Frame Errors
  note: Total Frames
  note: FER
  note: Total RErrors
  note: Total RBits
  note: Residual BER
  Rx Signal : Inport  Port=1  LatchInput=off
  Tx Raw Bits : Inport  Port=2  LatchInput=off
  Tx Info Bits : Inport  Port=3  LatchInput=off
  Hop : Inport  Port=4  LatchInput=off  SampleTime=Slot_Ts
  Enable : EnablePort
  Access Code Fail : Subsystem
      settings: RTWFcnNameOpts=Auto  RTWFileNameOpts=Auto
  Access Code or HEC fail : Logic  Operator=OR  Inputs=2
  Constant1 : Constant  Value=1
  DeFrame : dspindex/Multiport Selector  rowsOrCols=Rows  idxCellArray="{  1:72, 73:126,127:366}"  idxErrMode=Clip Index
  FER : commsink2/Error Rate Calculation  N=0  st_delay=0  cp_mode=Entire frame  subframe=[]  PMode=Port  WsName=ErrorVec  RsMode2=off  stop=on  numErr=100  maxBits=1e6
  FER Display : Display
      settings: Format=short
  Frame Status Conversion1 : dspsigattribs/Frame Status Conversion  growRefPort=off  outframe=Sample-based
  GMSK Demodulate and frequency hop : Subsystem
      settings: RTWFcnNameOpts=Auto  RTWFileNameOpts=Auto
  HEC Fail : Subsystem
      settings: RTWFcnNameOpts=Auto  RTWFileNameOpts=Auto
  Header info FEC Decode : Subsystem
      settings: RTWFcnNameOpts=Auto  RTWFileNameOpts=Auto
  Mux : Mux  Inputs=3
  Not all bits  equal3 : Logic  Operator=NOT  Inputs=1
  One Zeros : Subsystem
      settings: RTWFcnNameOpts=Auto  RTWFileNameOpts=Auto
  Payload FEC Decode : Subsystem
      settings: RTWFcnNameOpts=Auto  RTWFileNameOpts=Auto
  Raw BER : commsink2/Error Rate Calculation  N=0  st_delay=0  cp_mode=Entire frame  subframe=[]  PMode=Port  WsName=ErrorVec  RsMode2=off  stop=off  numErr=100  maxBits=1e6
  Raw BER Display : Display
      settings: Format=short
  Residual BER Display : Display
      settings: Format=short
  Residual BER Subsystem : Subsystem  TreatAsAtomicUnit=on
      settings: RTWFcnNameOpts=Auto  RTWFileNameOpts=Auto
  Selector : Selector  InputType=Vector  ElementSrc=Internal  Elements=[1 4 7]  RowSrc=Internal  Rows=1  ColumnSrc=Internal  Columns=1  InputPortWidth=9
  Switch : Switch  Threshold=.5
  To Workspace : ToWorkspace  VariableName=BER_Results  SampleTime=-1  SaveFormat=Array
      settings: MaxDataPoints=1
  Rx Info Bits : Outport  Port=1  InitialOutput=0
  wires:
  Hop/1 -> GMSK Demodulate and frequency hop/2(Hop)
  Rx Signal/1 -> GMSK Demodulate and frequency hop/1(Rx Signal)
  Switch/1 -> Payload FEC Decode/1(Input Bits)
  Not all bits  equal3/1 -> [Frame_OK]  "Frame OK"
  Frame Status Conversion1/1 -> Not all bits  equal3/1, Switch/2
  HEC Fail/1(Out) -> Access Code or HEC fail/2
  Header info FEC Decode/1(Out) -> HEC Fail/1(In)  "Header Info"
  Access Code Fail/1(Out) -> Access Code or HEC fail/1
  Access Code or HEC fail/1 -> Frame Status Conversion1/1  "Frame not ok"
  DeFrame/2 -> Header info FEC Decode/1(In)  "Header"
  One Zeros/1(One Zeros) -> Switch/1
  DeFrame/1 -> Access Code Fail/1(In)  "Access Code"
  DeFrame/3 -> Switch/3  "Payload"
  Tx Info Bits/1 -> Residual BER Subsystem/1(In1)  "Tx Info Bits"
  [Rx_Info_Bits] -> Residual BER Subsystem/2(In2)
  Constant1/1 -> FER/1
  Selector/1 -> To Workspace/1
  Mux/1 -> Selector/1
  Raw BER/1 -> Raw BER Display/1, Mux/1
  Tx Raw Bits/1 -> Raw BER/1
  FER/1 -> FER Display/1, Mux/3
  [Frame_OK] -> FER/2, Residual BER Subsystem/Enable
  Residual BER Subsystem/1(Out1) -> Mux/2, Residual BER Display/1
  Payload FEC Decode/1(Decoded Bits) -> [Rx_Info_Bits], Rx Info Bits/1
  [Rx_Raw_Bits] -> Raw BER/2
  GMSK Demodulate and frequency hop/1(Rx Raw Bits) -> DeFrame/1, [Rx_Raw_Bits]

== system bluetooth_voice/AWGN/Subsystem/Add noise ==
  In1 : Inport  Port=1  LatchInput=off
  Action Port : ActionPort  InitializeStates=held  ActionType=else
  AWGN Channel1 : commchan2/AWGN Channel  seed=seed  noiseMode="Signal to noise ratio  (Es/No)"  EsNodB=EsNo  SNRdB=10  Ps=Power  Tsym=Symbol_Period  variance=1
  Contiguous Copy : dspsigattribs/Contiguous Copy
  Out1 : Outport  Port=1
  wires:
  In1/1 -> AWGN Channel1/1
  Contiguous Copy/1 -> Out1/1
  AWGN Channel1/1 -> Contiguous Copy/1

== system bluetooth_voice/AWGN/Subsystem/Pass Through ==
  In1 : Inport  Port=1  LatchInput=off
  Action Port : ActionPort  InitializeStates=held  ActionType=then
  Out1 : Outport  Port=1
  wires:
  In1/1 -> Out1/1

== system bluetooth_voice/Instrumentation/Subsystem/Marker ==
  Enable : EnablePort
  DSP Constant : dspsrcs3/DSP Constant  Value=.1*[ones(1,36600) zeros(1,62500-36600)]'  InterpretAs1D=off  SampleMode=Discrete  Ts=625e-6  FramebasedOutput=on
  Tx : Outport  Port=1  OutputWhenDisabled=reset  InitialOutput=0
  wires:
  DSP Constant/1 -> Tx/1

== system bluetooth_voice/Master Transmitter/CVSD Encode/Set any 0's to 1's ==
  In1 : Inport  Port=1  LatchInput=off
  If : If  NumInputs=1  IfExpression=u1 ==0  ShowElse=on
  Merge : Merge  Inputs=2  AllowUnequalInputPortWidths=off  InputPortOffsets=[]
  Pass through : Subsystem  TreatAsAtomicUnit=on
      settings: RTWFcnNameOpts=Auto  RTWFileNameOpts=Auto
  Set to 1 : Subsystem  TreatAsAtomicUnit=on
      settings: RTWFcnNameOpts=Auto  RTWFileNameOpts=Auto
  Out1 : Outport  Port=1
  wires:
  If/1 -> Set to 1/Action
  In1/1 -> Pass through/1(In1), If/1
  If/2 -> Pass through/Action
  Set to 1/1(1) -> Merge/1
  Pass through/1(Out1=In1) -> Merge/2
  Merge/1 -> Out1/1  "y"

== system bluetooth_voice/Master Transmitter/CVSD Encode/Update accum ==
  stepsize(n+1) : Inport  Port=1  LatchInput=off
  y : Inport  Port=2  LatchInput=off
  accum(n) : Inport  Port=3  LatchInput=off
  Gain : Gain  Gain=accum_decay  Multiplication=Element-wise(K.*u)  SaturateOnIntegerOverflow=on
  Product : Product  Inputs=2  Multiplication=Element-wise(.*)  SaturateOnIntegerOverflow=on
  Saturation : Saturate  UpperLimit=pos_accum_max  LowerLimit=neg_accum_max  LinearizeAsGain=on
  Sum1 : Sum  Inputs=|++  SaturateOnIntegerOverflow=on
  accum(n+1) : Outport  Port=1
  wires:
  Gain/1 -> Saturation/1
  Product/1 -> Sum1/1  "y*stepsize"
  Sum1/1 -> Gain/1
  stepsize(n+1)/1 -> Product/1
  y/1 -> Product/2
  accum(n)/1 -> Sum1/2
  Saturation/1 -> accum(n+1)/1

== system bluetooth_voice/Master Transmitter/CVSD Encode/Update runner ==
  y : Inport  Port=1  LatchInput=off
  runner(n) : Inport  Port=2  LatchInput=off
  Bitwise Logical Operator : simulink3/Math/Bitwise Logical Operator  Operator=AND  Operand2=15
  Data Type Conversion : DataTypeConversion  DataType=uint16  SaturateOnIntegerOverflow=on
  Data Type Conversion1 : DataTypeConversion  DataType=double  SaturateOnIntegerOverflow=on
  Fcn : Fcn  Expr=u==1
  Gain : Gain  Gain=2  Multiplication=Element-wise(K.*u)  SaturateOnIntegerOverflow=on
  Sum1 : Sum  Inputs=|++  SaturateOnIntegerOverflow=on
  runner(n+1) : Outport  Port=1
  wires:
  Gain/1 -> Sum1/2  "2*runner"
  Fcn/1 -> Sum1/1  "y==1"
  Sum1/1 -> Data Type Conversion/1
  Data Type Conversion/1 -> Bitwise Logical Operator/1
  y/1 -> Fcn/1
  Bitwise Logical Operator/1 -> Data Type Conversion1/1
  runner(n)/1 -> Gain/1
  Data Type Conversion1/1 -> runner(n+1)/1

== system bluetooth_voice/Master Transmitter/CVSD Encode/Update stepsize ==
  runner(n+1) : Inport  Port=1  LatchInput=off
  stepsize(n) : Inport  Port=2  LatchInput=off
  If : If  NumInputs=1  IfExpression=(u1 == 0) | (u1== 15)  ShowElse=on
  Merge1 : Merge  Inputs=2  AllowUnequalInputPortWidths=off  InputPortOffsets=[]
  Update : Subsystem  TreatAsAtomicUnit=on
      settings: RTWFcnNameOpts=Auto  RTWFileNameOpts=Auto
  Update1 : Subsystem  TreatAsAtomicUnit=on
      settings: RTWFcnNameOpts=Auto  RTWFileNameOpts=Auto
  stepsize(n+1) : Outport  Port=1
  wires:
  If/2 -> Update1/Action
  If/1 -> Update/Action  "(runner == 0) | (runner == 15)"
  Update/1(stepsize(n+1)) -> Merge1/1
  stepsize(n)/1 -> Update1/1(stepsize), Update/1(stepsize)
  Update1/1(stepsize(n+1)) -> Merge1/2
  runner(n+1)/1 -> If/1
  Merge1/1 -> stepsize(n+1)/1

== system bluetooth_voice/Master Transmitter/Encode and modulate/Bluetooth HEC Generator ==
  In1 : Inport  Port=1  LatchInput=off
  Frame Status Conversion : dspsigattribs/Frame Status Conversion  growRefPort=off  outframe=Sample-based
  Frame Status Conversion1 : dspsigattribs/Frame Status Conversion  growRefPort=on  outframe=Sample-based
  S-Function Builder : S-Function  AncestorBlock=|  FunctionName=scomdemohecgen  Parameters=uap  PortCounts=[]  SFunctionModules=scomdemohecgen_wrapper
      | simulink3/Functions
      | & Tables/Basic S-Function
      | Builder
      mask init:
      | val = [[.9  0.75 0.75 1 1 .9 .9 1]',[1 1 0.75 0.75 .9 .9 1 .9]'];
      | sys = get_param(gcb,'FunctionName');
      settings: CopyFcn=set_param(gcb,'LinkStatus','none')  OpenFcn=sfunctionwizard(gcbh)
      mask Display:
      | plot(val(:,1),val(:,2))
      | disp(sys)
  Out1 : Outport  Port=1
  wires:
  Frame Status Conversion/1 -> S-Function Builder/1
  Frame Status Conversion1/1 -> Out1/1
  In1/1 -> Frame Status Conversion1/2, Frame Status Conversion/1
  S-Function Builder/1 -> Frame Status Conversion1/1

== system bluetooth_voice/Master Transmitter/Encode and modulate/GMSK Modulate and frequency hop ==
  Tx Raw Bits : Inport  Port=1  LatchInput=off
  Hop : Inport  Port=2  LatchInput=off
  Frame Status Conversion : dspsigattribs/Frame Status Conversion  growRefPort=off  outframe=Frame-based
  GFSK Modulation : commdigbbndcpm2/CPM Modulator Baseband  Mnum=2  inputType=Bit  mappingType=Binary  modIdx=0.32  pulseShape=Gaussian  BT=0.5  rollOff=0.2  pulseLength=1  preHistory=1  phaseOffset=0  samplesPerSymbol=100
  "Generate 79 possible carriers -39MHz to 39MHz " : commdigbbndfm2/M-FSK Modulator Baseband  M=79  InType=Integer  Enc=Binary  freqSep=1e6  phaseType=Continuous  numSamp=6.25e4
  Mask to turn off transmitter after data finished : Gain  Gain=[ones(36600,1);zeros(62500-36600,1)]  Multiplication=Element-wise(K.*u)  SaturateOnIntegerOverflow=on
  Product3 : Product  Inputs=2  Multiplication=Element-wise(.*)  SaturateOnIntegerOverflow=on
  Set to 0dBm : dspmathops/dB Gain  Gain=g  dB=-30  intype=Amplitude
  Zero Pad to fill slot : dspsigops/Zero Pad  zpadAlong=Columns  numOutRows=625  numOutCols=1  trunc_flag=None
  Tx SIgnal : Outport  Port=1
  wires:
  Product3/1 -> Mask to turn off transmitter after data finished/1
  Mask to turn off transmitter after data finished/1 -> Set to 0dBm/1
  Zero Pad to fill slot/1 -> GFSK Modulation/1
  Frame Status Conversion/1 -> "Generate 79 possible carriers -39MHz to 39MHz "/1
  "Generate 79 possible carriers -39MHz to 39MHz "/1 -> Product3/2
  GFSK Modulation/1 -> Product3/1
  Tx Raw Bits/1 -> Zero Pad to fill slot/1
  Set to 0dBm/1 -> Tx SIgnal/1
  Hop/1 -> Frame Status Conversion/1

== system bluetooth_voice/Master Transmitter/Encode and modulate/Header Info ==
  Header3 : dspsrcs3/DSP Constant  Value=Slave_Address  InterpretAs1D=off  SampleMode=Discrete  Ts=Slot_Ts  FramebasedOutput=on
  Header4 : dspsrcs3/DSP Constant  Value=Packet_Type  InterpretAs1D=off  SampleMode=Discrete  Ts=Slot_Ts  FramebasedOutput=on
  Header5 : dspsrcs3/DSP Constant  Value=Flow_Control  InterpretAs1D=off  SampleMode=Discrete  Ts=Slot_Ts  FramebasedOutput=on
  Header6 : dspsrcs3/DSP Constant  Value=ARQ  InterpretAs1D=off  SampleMode=Discrete  Ts=Slot_Ts  FramebasedOutput=on
  Header7 : dspsrcs3/DSP Constant  Value=Sequence  InterpretAs1D=off  SampleMode=Discrete  Ts=Slot_Ts  FramebasedOutput=on
  Matrix Concatenation1 : simulink3/Signals & Systems/Matrix Concatenation  numInports=5  catMethod=Vertical
  Out : Outport  Port=1
  wires:
  Header3/1 -> Matrix Concatenation1/1  "Slave address"
  Header4/1 -> Matrix Concatenation1/2  "Packet type"
  Header5/1 -> Matrix Concatenation1/3  "Flow control"
  Header6/1 -> Matrix Concatenation1/4  "ARQ"
  Header7/1 -> Matrix Concatenation1/5  "Sequence"
  Matrix Concatenation1/1 -> Out/1  "Header Info"

== system bluetooth_voice/Master Transmitter/Payload FEC Encode/FEC HV1 ==
  In : Inport  Port=1  LatchInput=off
  Enable : EnablePort
  Buffer : dspbuff3/Buffer  N=80  V=0  ic=0
  FEC : dspsigops/Repeat  N=3  ic=0  mode=Maintain input frame rate
  Sample Tx_Ts1 : ZeroOrderHold  SampleTime=Slot_Ts
  Sample Tx_Ts2 : ZeroOrderHold  SampleTime=Slot_Ts
  Zero Pad : dspsigops/Zero Pad  zpadAlong=Columns  numOutRows=240  numOutCols=1  trunc_flag=None
  FEC'd : Outport  Port=1
  Bits : Outport  Port=2
  wires:
  In/1 -> Buffer/1
  FEC/1 -> Sample Tx_Ts1/1
  Sample Tx_Ts1/1 -> FEC'd/1
  Zero Pad/1 -> Sample Tx_Ts2/1
  Sample Tx_Ts2/1 -> Bits/1
  Buffer/1 -> FEC/1, Zero Pad/1

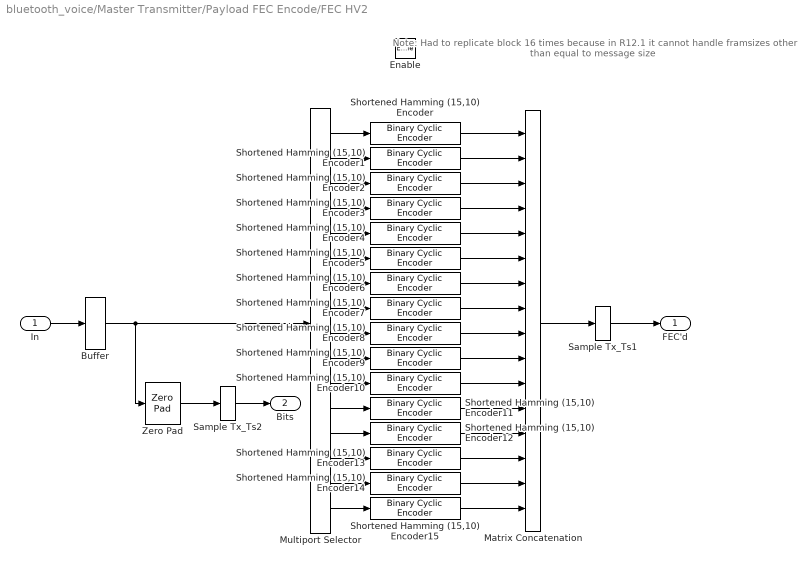
== system bluetooth_voice/Master Transmitter/Payload FEC Encode/FEC HV2 ==
  note: Note: Had to replicate block 16 times
      | because in R12.1 it cannot handle framsizes
      | other than equal to message size
  In : Inport  Port=1  LatchInput=off
  Enable : EnablePort
  Buffer : dspbuff3/Buffer  N=160  V=0  ic=0
  Matrix Concatenation : simulink3/Signals & Systems/Matrix Concatenation  numInports=16  catMethod=Vertical
  Multiport Selector : dspindex/Multiport Selector  rowsOrCols=Rows  idxCellArray={ 1:10, 11:20,21:30,31:40,41:50,51:60,61:70,71:80,81:90,91:100,101:110,111:120,121:130,131:140,141:150,151:160}  idxErrMode=Clip Index
  Sample Tx_Ts1 : ZeroOrderHold  SampleTime=Slot_Ts
  Sample Tx_Ts2 : ZeroOrderHold  SampleTime=Slot_Ts
  Shortened Hamming (15,10) Encoder{,1..15} (16 alike) : commblkcod2/Binary Cyclic Encoder  n=15  p=[1 1 0 1 0 1]
  Zero Pad : dspsigops/Zero Pad  zpadAlong=Columns  numOutRows=240  numOutCols=1  trunc_flag=None
  FEC'd : Outport  Port=1
  Bits : Outport  Port=2
  wires:
  In/1 -> Buffer/1
  Buffer/1 -> Multiport Selector/1, Zero Pad/1
  Multiport Selector/1 -> Shortened Hamming (15,10) Encoder/1
  Multiport Selector/2 -> Shortened Hamming (15,10) Encoder1/1
  Multiport Selector/3 -> Shortened Hamming (15,10) Encoder2/1
  Multiport Selector/4 -> Shortened Hamming (15,10) Encoder3/1
  Multiport Selector/5 -> Shortened Hamming (15,10) Encoder4/1
  Multiport Selector/6 -> Shortened Hamming (15,10) Encoder5/1
  Multiport Selector/7 -> Shortened Hamming (15,10) Encoder6/1
  Multiport Selector/8 -> Shortened Hamming (15,10) Encoder7/1
  Multiport Selector/9 -> Shortened Hamming (15,10) Encoder8/1
  Multiport Selector/10 -> Shortened Hamming (15,10) Encoder9/1
  Multiport Selector/11 -> Shortened Hamming (15,10) Encoder10/1
  Multiport Selector/12 -> Shortened Hamming (15,10) Encoder11/1
  Multiport Selector/13 -> Shortened Hamming (15,10) Encoder12/1
  Multiport Selector/14 -> Shortened Hamming (15,10) Encoder13/1
  Multiport Selector/15 -> Shortened Hamming (15,10) Encoder14/1
  Multiport Selector/16 -> Shortened Hamming (15,10) Encoder15/1
  Shortened Hamming (15,10) Encoder/1 -> Matrix Concatenation/1
  Shortened Hamming (15,10) Encoder1/1 -> Matrix Concatenation/2
  Shortened Hamming (15,10) Encoder2/1 -> Matrix Concatenation/3
  Shortened Hamming (15,10) Encoder3/1 -> Matrix Concatenation/4
  Shortened Hamming (15,10) Encoder4/1 -> Matrix Concatenation/5
  Shortened Hamming (15,10) Encoder5/1 -> Matrix Concatenation/6
  Shortened Hamming (15,10) Encoder6/1 -> Matrix Concatenation/7
  Shortened Hamming (15,10) Encoder7/1 -> Matrix Concatenation/8
  Shortened Hamming (15,10) Encoder8/1 -> Matrix Concatenation/9
  Shortened Hamming (15,10) Encoder9/1 -> Matrix Concatenation/10
  Shortened Hamming (15,10) Encoder10/1 -> Matrix Concatenation/11
  Shortened Hamming (15,10) Encoder11/1 -> Matrix Concatenation/12
  Shortened Hamming (15,10) Encoder12/1 -> Matrix Concatenation/13
  Shortened Hamming (15,10) Encoder13/1 -> Matrix Concatenation/14
  Shortened Hamming (15,10) Encoder14/1 -> Matrix Concatenation/15
  Shortened Hamming (15,10) Encoder15/1 -> Matrix Concatenation/16
  Matrix Concatenation/1 -> Sample Tx_Ts1/1
  Zero Pad/1 -> Sample Tx_Ts2/1
  Sample Tx_Ts1/1 -> FEC'd/1
  Sample Tx_Ts2/1 -> Bits/1

== system bluetooth_voice/Master Transmitter/Payload FEC Encode/FEC HV3 (None) ==
  In : Inport  Port=1  LatchInput=off
  Enable : EnablePort
  Buffer : dspbuff3/Buffer  N=240  V=0  ic=0
  Sample Tx_Ts1 : ZeroOrderHold  SampleTime=Slot_Ts
  Sample Tx_Ts2 : ZeroOrderHold  SampleTime=Slot_Ts
  FEC'd : Outport  Port=1
  Bits : Outport  Port=2
  wires:
  In/1 -> Buffer/1
  Sample Tx_Ts1/1 -> FEC'd/1
  Sample Tx_Ts2/1 -> Bits/1
  Buffer/1 -> Sample Tx_Ts1/1, Sample Tx_Ts2/1

== system bluetooth_voice/Slave Receiver/CVSD Decode/Update accum ==
  stepsize(n+1) : Inport  Port=1  LatchInput=off
  u : Inport  Port=2  LatchInput=off
  accum(n) : Inport  Port=3  LatchInput=off
  Gain : Gain  Gain=accum_decay  Multiplication=Element-wise(K.*u)  SaturateOnIntegerOverflow=on
  Product : Product  Inputs=2  Multiplication=Element-wise(.*)  SaturateOnIntegerOverflow=on
  Saturation : Saturate  UpperLimit=pos_accum_max  LowerLimit=neg_accum_max  LinearizeAsGain=on
  Sum1 : Sum  Inputs=|++  SaturateOnIntegerOverflow=on
  accum(n+1) : Outport  Port=1
  wires:
  Product/1 -> Sum1/1  "y*stepsize"
  Sum1/1 -> Gain/1
  stepsize(n+1)/1 -> Product/1
  u/1 -> Product/2
  accum(n)/1 -> Sum1/2
  Gain/1 -> Saturation/1
  Saturation/1 -> accum(n+1)/1

== system bluetooth_voice/Slave Receiver/CVSD Decode/Update runner ==
  u : Inport  Port=1  LatchInput=off
  runner(n) : Inport  Port=2  LatchInput=off
  Bitwise Logical Operator : simulink3/Math/Bitwise Logical Operator  Operator=AND  Operand2=15
  Data Type Conversion : DataTypeConversion  DataType=uint16  SaturateOnIntegerOverflow=on
  Data Type Conversion1 : DataTypeConversion  DataType=double  SaturateOnIntegerOverflow=on
  Fcn : Fcn  Expr=u==1
  Gain : Gain  Gain=2  Multiplication=Element-wise(K.*u)  SaturateOnIntegerOverflow=on
  Sum1 : Sum  Inputs=|++  SaturateOnIntegerOverflow=on
  runner(n+1) : Outport  Port=1
  wires:
  Gain/1 -> Sum1/2  "2*runner"
  Fcn/1 -> Sum1/1  "y==1"
  Sum1/1 -> Data Type Conversion/1
  Data Type Conversion/1 -> Bitwise Logical Operator/1
  u/1 -> Fcn/1
  Bitwise Logical Operator/1 -> Data Type Conversion1/1
  runner(n)/1 -> Gain/1
  Data Type Conversion1/1 -> runner(n+1)/1

== system bluetooth_voice/Slave Receiver/CVSD Decode/Update stepsize ==
  runner(n+1) : Inport  Port=1  LatchInput=off
  stepsize(n) : Inport  Port=2  LatchInput=off
  If : If  NumInputs=1  IfExpression=(u1 == 0) | (u1== 15)  ShowElse=on
  Merge1 : Merge  Inputs=2  AllowUnequalInputPortWidths=off  InputPortOffsets=[]
  Update : Subsystem  TreatAsAtomicUnit=on
      settings: RTWFcnNameOpts=Auto  RTWFileNameOpts=Auto
  Update1 : Subsystem  TreatAsAtomicUnit=on
      settings: RTWFcnNameOpts=Auto  RTWFileNameOpts=Auto
  stepsize(n+1) : Outport  Port=1
  wires:
  If/1 -> Update/Action  "(runner == 0) | (runner == 15)"
  Update/1(stepsize(n+1)) -> Merge1/1
  stepsize(n)/1 -> Update1/1(stepsize), Update/1(stepsize)
  If/2 -> Update1/Action
  Update1/1(stepsize(n+1)) -> Merge1/2
  runner(n+1)/1 -> If/1
  Merge1/1 -> stepsize(n+1)/1

== system bluetooth_voice/Slave Receiver/Demodulate and decode/Access Code Fail ==
  In : Inport  Port=1  LatchInput=off
  Access Code : dspsrcs3/DSP Constant  Value=Access_Code  InterpretAs1D=off  SampleMode=Discrete  Ts=Slot_Ts  FramebasedOutput=on
  Constant : Constant  Value=57
  Less than  57 bits good : RelationalOperator  Operator=<
  Relational Operator : RelationalOperator  Operator===
  Strip of preamble  and trailer : Selector  InputType=Vector  ElementSrc=Internal  Elements=[5:68]  RowSrc=Internal  Rows=1  ColumnSrc=Internal  Columns=1  InputPortWidth=72
  Strip of preamble  and trailer1 : Selector  InputType=Vector  ElementSrc=Internal  Elements=[5:68]  RowSrc=Internal  Rows=1  ColumnSrc=Internal  Columns=1  InputPortWidth=72
  Total correct bits : Sum  Inputs=1  SaturateOnIntegerOverflow=on
  Out : Outport  Port=1
  wires:
  Less than  57 bits good/1 -> Out/1
  In/1 -> Strip of preamble  and trailer1/1
  Constant/1 -> Less than  57 bits good/2
  Total correct bits/1 -> Less than  57 bits good/1
  Strip of preamble  and trailer/1 -> Relational Operator/1
  Strip of preamble  and trailer1/1 -> Relational Operator/2
  Relational Operator/1 -> Total correct bits/1
  Access Code/1 -> Strip of preamble  and trailer/1
